simulink model "fig2_19bx"  (R2014a)
settings: Solver=ode45  StartTime=0.0  StopTime=10.0  MaxStep=.05  MinStep=.01  RelTol=1e-3
settings Model: Creator=Office Depot  LastModifiedBy=D
settings SolverCC: InitialStep=.01
settings DataIOCC: SignalLoggingSaveFormat=ModelDataLogs
settings OptimizationCC: ExpressionDepthLimit=2147483647  InitFltsAndDblsToZero=on
settings DebuggingCC: UnderspecifiedInitializationDetection=Classic  FcnCallInpInsideContextMsg=UseLocalSettings  StateNameClashWarn=warning  StrictBusMsg=Warning
settings GRTTargetCC: CombineOutputUpdateFcns=off  GRTInterface=on

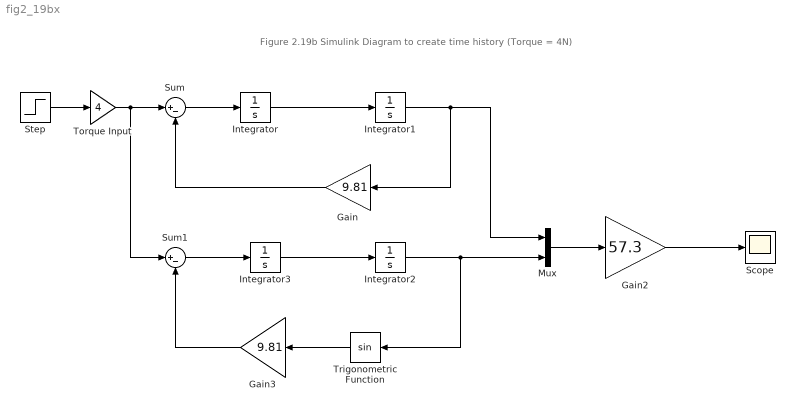
== system fig2_19bx ==
  note: Figure 2.19b Simulink Diagram to create time history (Torque = 4N)
  Gain : Gain  Gain=9.81
  Gain2 : Gain  Gain=57.3
  Gain3 : Gain  Gain=9.81
  Integrator{,1..3} (4 alike) : Integrator
  Mux : Mux  Inputs=2
  Scope : Scope
  Step : Step  Time=0  SampleTime=0
  Sum : Sum  Inputs=|+-
  Sum1 : Sum  Inputs=|+-
  Torque Input : Gain  Gain=4
  Trigonometric Function : Trigonometry
  wires:
  Integrator/1 -> Integrator1/1
  Integrator1/1 -> Mux/1, Gain/1
  Sum/1 -> Integrator/1
  Gain/1 -> Sum/2
  Step/1 -> Torque Input/1
  Torque Input/1 -> Sum/1, Sum1/1
  Integrator2/1 -> Mux/2, Trigonometric Function/1
  Integrator3/1 -> Integrator2/1
  Sum1/1 -> Integrator3/1
  Gain2/1 -> Scope/1
  Trigonometric Function/1 -> Gain3/1
  Gain3/1 -> Sum1/2
  Mux/1 -> Gain2/1
